simulink model "ndu_PID"  (R2021a)
settings: Solver=VariableStepAuto  StartTime=0.0  StopTime=250  RelTol=1e-3
model workspace (MAT data in the model file):
  J1 = 0.1
  K1 = 0.1
  K2 = 0.0015625
libraries: pid_lib x1
settings Model: Creator=Jurica Vučković  LastModifiedBy=Jurica Vučković
settings DataIOCC: ExternalInput=ts  OutputSaveName=w2

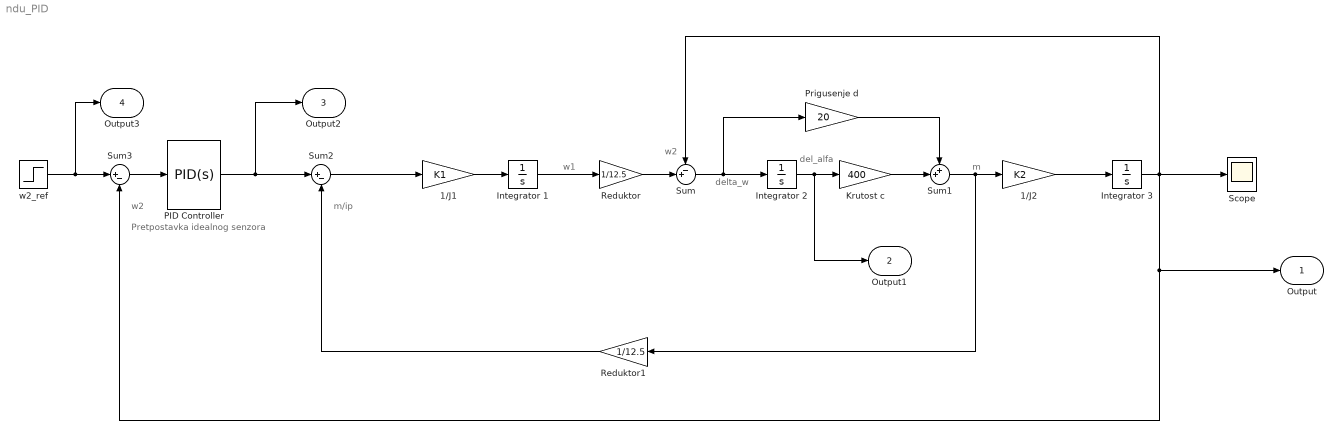
== system ndu_PID ==
  note: Pretpostavka idealnog senzora
  note: w2
  note: m/ip
  note: m
  note: del_alfa
  note: w2
  note: delta_w
  note: w1
  1/J1 : Gain  Gain=K1
  1/J2 : Gain  Gain=K2
  Integrator 1 : Integrator
  Integrator 2 : Integrator  LimitOutput=on  UpperSaturationLimit=0.2  LowerSaturationLimit=-0.2
  Integrator 3 : Integrator
  Krutost c : Gain  Gain=400
  PID Controller : pid_lib/PID Controller  Controller=PID  Form=Parallel  TimeDomain=Continuous-time  UseExternalTs=off  SampleTime=-1  IntegratorMethod=Forward Euler  FilterMethod=Forward Euler  ControllerParametersSource=internal  P=6.14475808574894  I=0.00185277865975379  D=-26.834616265965  UseFilter=on  N=0.187689822698302  TunerSelectOption=Transfer Function Based (PID Tuner App)  InitialConditionSource=internal  InitialConditionForIntegrator=0  InitialConditionForFilter=0  DifferentiatorICPrevScaledInput=0  ExternalReset=none  TrackingMode=off  Kt=1  LimitOutput=on  SatLimitsSource=internal  UpperSaturationLimit=200  LowerSaturationLimit=-200  LinearizeAsGain=off  AntiWindupMode=none  Kb=1  POutMin=[]  POutMax=[]  IOutMin=[]  IOutMax=[]  DOutMin=[]  DOutMax=[]  NOutMin=[]  NOutMax=[]  SumOutMin=[]  SumOutMax=[]  SaturationOutMin=[]  SaturationOutMax=[]  PParamMin=[]  PParamMax=[]  IParamMin=[]  IParamMax=[]  DParamMin=[]  DParamMax=[]  NParamMin=[]  NParamMax=[]  KbParamMin=[]  KbParamMax=[]  KtParamMin=[]  KtParamMax=[]  KbOutMin=[]  KbOutMax=[]  KtOutMin=[]  KtOutMax=[]  IntegratorOutMin=[]  IntegratorOutMax=[]  FilterOutMin=[]  FilterOutMax=[]  SumI1OutMin=[]  SumI1OutMax=[]  SumI2OutMin=[]  SumI2OutMax=[]  SumI3OutMin=[]  SumI3OutMax=[]  SumI4OutMin=[]  SumI4OutMax=[]  SumDOutMin=[]  SumDOutMax=[]  DifferentiatorOutMin=[]  DifferentiatorOutMax=[]  FilterDiffOutCoefMin=[]  FilterDiffOutCoefMax=[]  ReciprocalOutMin=[]  ReciprocalOutMax=[]  SumDenOutMin=[]  SumDenOutMax=[]  SumNumOutMin=[]  SumNumOutMax=[]  DivideOutMin=[]  DivideOutMax=[]  UdiffTsProdOutMin=[]  UdiffTsProdOutMax=[]  NTsProdOutMin=[]  NTsProdOutMax=[]  UintegralTsProdOutMin=[]  UintegralTsProdOutMax=[]  UngainTsProdOutMin=[]  UngainTsProdOutMax=[]  IntegratorContinuousStateAttributes=''  IntegratorStateMustResolveToSignalObject=off  IntegratorRTWStateStorageClass=Auto  FilterContinuousStateAttributes=''  FilterStateMustResolveToSignalObject=off  FilterRTWStateStorageClass=Auto  ParallelPVariant=InternalParameters  IdealPVariant=Disabled  IVariant=InternalParameters  DVariant=InternalParameters  IntegratorVariant=Continuous  SatVariant=Enabled  AWVariant=Passthrough  PCopyVariant=Disabled  TRVariant=Disabled  FdbkBlocksVariant=Forward  IdealPFdbkVariant=Disabled  SatFdbkVariant=Disabled  DerivativeFilterVariant=ContFilter  NVariant=InternalParameters  NCopyVariant=Disabled  FilterICVariant=InternalICsFilter  IntegratorICVariant=InternalICs  ExternalResetVariant=Disabled  TRSumVariant=Passthrough  SumFdbkVariant=Disabled  SumVariant=Sum_PID  TsampFilterVariant=InternalTs  TsampNgainVariant=Passthrough  TsampIntegralVariant=Passthrough  ExternalSaturationOutDataTypeStr=Inherit: Same as second input
  Prigusenje d : Gain  Gain=20
  Reduktor : Gain  Gain=1/12.5
  Reduktor1 : Gain  Gain=1/12.5
  Scope : Scope
  Sum : Sum  Inputs=-+|
  Sum1 : Sum  Inputs=++|
  Sum2 : Sum  Inputs=|+-
  Sum3 : Sum  Inputs=|+-
  w2_ref : Step  After=30  SampleTime=1
  Output : Outport  SignalName=w2
  Output1 : Outport  Port=2  SignalName=delta_alfa
  Output2 : Outport  Port=3  SignalName=m1
  Output3 : Outport  Port=4  SignalName=w2,ref
  wires:
  1/J1/1 -> Integrator 1/1
  Integrator 1/1 -> Reduktor/1
  Reduktor/1 -> Sum/2
  Krutost c/1 -> Sum1/2
  Sum/1 -> Prigusenje d/1, Integrator 2/1
  Prigusenje d/1 -> Sum1/1
  1/J2/1 -> Integrator 3/1
  Integrator 3/1 -> Sum3/2, Output/1, Scope/1, Sum/1
  Sum1/1 -> Reduktor1/1, 1/J2/1
  Reduktor1/1 -> Sum2/2
  Sum2/1 -> 1/J1/1
  w2_ref/1 -> Output3/1, Sum3/1
  Sum3/1 -> PID Controller/1
  Integrator 2/1 -> Output1/1, Krutost c/1
  PID Controller/1 -> Output2/1, Sum2/1
